simulink model "unfinished_total"  (Simulink 7.9)
settings: Solver=ode3  StartTime=0.0  StopTime=100.0  RelTol=1e-3
undefined symbols (not defined in the file or in its folder): DiscIntNeverNeededParam
libraries: dspsrcs4 x1, simulink x1
settings Model: Creator=dAN  LastModifiedBy=dAN

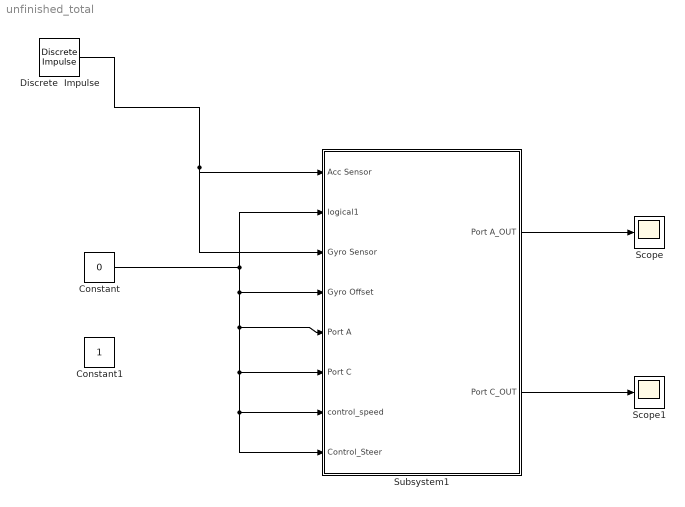
== system unfinished_total ==
  Constant : Constant  Value=0
  Constant1 : Constant
  Discrete  Impulse : dspsrcs4/Discrete  Impulse  Delay=5  SampleTime=1  FrameSample=1  dataType=double  isSigned=on  wordLen=16  udDataType=sfix(16)  fracBitsMode=Best precision  numFracBits=15  OutDataTypeStr=double  LastOutDataTypeStr=double
  Scope : Scope
  Scope1 : Scope
      settings: TimeRange=10
  Subsystem1 : Subsystem
  wires:
  Subsystem1/2(Port C_OUT) -> Scope1/1
  Subsystem1/1(Port A_OUT) -> Scope/1
  Constant/1 -> Subsystem1/4(Gyro Offset), Subsystem1/5(Port A), Subsystem1/7(control_speed), Subsystem1/8(Control_Steer), Subsystem1/6(Port C), Subsystem1/2(logical1)
  Discrete  Impulse/1 -> Subsystem1/1(Acc Sensor), Subsystem1/3(Gyro Sensor)

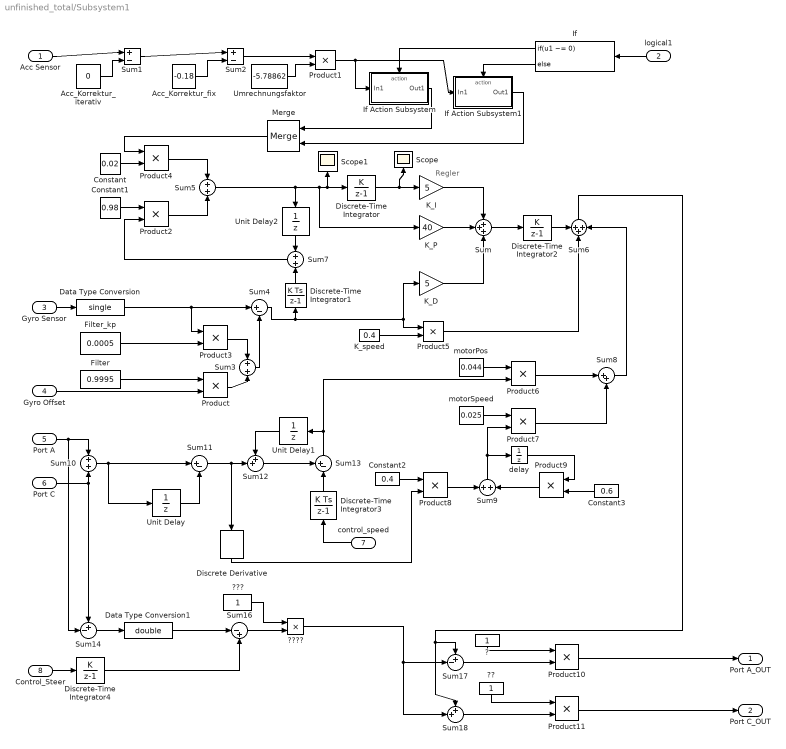
== system unfinished_total/Subsystem1 ==
  note: Regler
  Acc Sensor : Inport
  logical1 : Inport  Port=2
  Gyro Sensor : Inport  Port=3
  Gyro Offset : Inport  Port=4
  Port A : Inport  Port=5
  Port C : Inport  Port=6
  control_speed : Inport  Port=7
  Control_Steer : Inport  Port=8
  "?" : Constant
  "??" : Constant
  "???" : Constant
  "????" : Product  RndMeth=Zero
  Acc_Korrektur_fix : Constant  Value=-0.18
  Acc_Korrektur_iterativ : Constant  Value=0
  Constant : Constant  Value=0.02
  Constant1 : Constant  Value=0.98
  Constant2 : Constant  Value=0.4
  Constant3 : Constant  Value=0.6
  Data Type Conversion : DataTypeConversion  OutDataTypeStr=single  ConvertRealWorld=Stored Integer (SI)
  Data Type Conversion1 : DataTypeConversion  OutDataTypeStr=double  ConvertRealWorld=Stored Integer (SI)
  Discrete Derivative : simulink/Discrete/Discrete Derivative  gainval=1.0  ICPrevScaledInput=0.0  InputProcessing=Inherited  OutMin=[]  OutMax=[]  OutDataType=fixdt(1, 16)  OutScaling=2^-10  DoSatur=off
  Discrete-Time Integrator : DiscreteIntegrator  IntegratorMethod=Accumulation: Forward Euler  ICPrevOutput=DiscIntNeverNeededParam  ICPrevScaledInput=DiscIntNeverNeededParam
  Discrete-Time Integrator1 : DiscreteIntegrator  ICPrevOutput=DiscIntNeverNeededParam  ICPrevScaledInput=DiscIntNeverNeededParam
  Discrete-Time Integrator2 : DiscreteIntegrator  IntegratorMethod=Accumulation: Forward Euler  ICPrevOutput=DiscIntNeverNeededParam  ICPrevScaledInput=DiscIntNeverNeededParam
  Discrete-Time Integrator3 : DiscreteIntegrator  ICPrevOutput=DiscIntNeverNeededParam  ICPrevScaledInput=DiscIntNeverNeededParam
  Discrete-Time Integrator4 : DiscreteIntegrator  IntegratorMethod=Accumulation: Forward Euler  ICPrevOutput=DiscIntNeverNeededParam  ICPrevScaledInput=DiscIntNeverNeededParam
  Filter : Constant  Value=0.9995
  Filter_kp : Constant  Value=0.0005
  If : If  IfExpression=u1 ~= 0
  If Action Subsystem : Subsystem  TreatAsAtomicUnit=on
  If Action Subsystem1 : Subsystem  TreatAsAtomicUnit=on
  K_D : Gain  Gain=5
  K_I : Gain  Gain=5
  K_P : Gain  Gain=40
  K_speed : Constant  Value=0.4
  Merge : Merge
  Product{,1..11} (12 alike) : Product  RndMeth=Zero
  Scope : Scope
      settings: SaveName=ScopeData2
  Scope1 : Scope
      settings: SaveName=ScopeData3
  Sum : Sum  Inputs=+++
  Sum{1..2,4,11} (4 alike) : Sum  Inputs=|+-
  Sum{3,5,7,9..10} (5 alike) : Sum  Inputs=+|+
  Sum12 : Sum  Inputs=++|
  Sum13 : Sum  Inputs=+-|
  Sum14 : Sum  Inputs=+-|
  Sum16 : Sum  Inputs=|-+
  Sum17 : Sum  Inputs=+-|
  Sum18 : Sum  Inputs=++|
  Sum6 : Sum  Inputs=+++
  Sum8 : Sum  Inputs=|++
  Umrechnungsfaktor : Constant  Value=-5.78862
  Unit Delay : UnitDelay  SampleTime=-1
  Unit Delay1 : UnitDelay  SampleTime=-1
  Unit Delay2 : UnitDelay  SampleTime=-1
  delay : UnitDelay  SampleTime=-1
  motorPos : Constant  Value=0.044
  motorSpeed : Constant  Value=0.025
  Port A_OUT : Outport
  Port C_OUT : Outport  Port=2
  wires:
  K_I/1 -> Sum/1
  K_P/1 -> Sum/2
  K_D/1 -> Sum/3
  Discrete-Time Integrator/1 -> K_I/1, Scope/1
  Gyro Offset/1 -> Product/2
  Filter/1 -> Product/1
  Acc Sensor/1 -> Sum1/1
  Acc_Korrektur_iterativ/1 -> Sum1/2
  Acc_Korrektur_fix/1 -> Sum2/2
  Sum1/1 -> Sum2/1
  Umrechnungsfaktor/1 -> Product1/2
  Sum2/1 -> Product1/1
  Gyro Sensor/1 -> Data Type Conversion/1
  Data Type Conversion/1 -> Product3/1, Sum4/1
  Filter_kp/1 -> Product3/2
  Product3/1 -> Sum3/1
  Product/1 -> Sum3/2
  Sum3/1 -> Sum4/2
  Constant/1 -> Product4/2
  Constant1/1 -> Product2/1
  Product4/1 -> Sum5/1
  Product2/1 -> Sum5/2
  Sum7/1 -> Product2/2
  Sum5/1 -> K_P/1, Discrete-Time Integrator/1, Scope1/1, Unit Delay2/1
  Sum/1 -> Discrete-Time Integrator2/1
  K_speed/1 -> Product5/2
  Discrete-Time Integrator2/1 -> Sum6/1
  Product5/1 -> Sum6/2
  Sum8/1 -> Sum6/3
  motorPos/1 -> Product6/1
  Product6/1 -> Sum8/1
  Product7/1 -> Sum8/2
  motorSpeed/1 -> Product7/1
  Product8/1 -> Sum9/1
  Sum9/1 -> Product7/2, delay/1
  Port A/1 -> Sum10/1, Sum14/2
  Port C/1 -> Sum10/2, Sum14/1
  Sum10/1 -> Sum11/1, Unit Delay/1
  Unit Delay/1 -> Sum11/2
  Sum13/1 -> Product6/2, Unit Delay1/1
  Sum12/1 -> Sum13/1
  Sum11/1 -> Sum12/2, Discrete Derivative/1
  Discrete-Time Integrator3/1 -> Sum13/2
  control_speed/1 -> Discrete-Time Integrator3/1
  Product9/1 -> Sum9/2
  Constant3/1 -> Product9/2
  Constant2/1 -> Product8/1
  Discrete Derivative/1 -> Product8/2
  Sum14/1 -> Data Type Conversion1/1
  Control_Steer/1 -> Discrete-Time Integrator4/1
  Data Type Conversion1/1 -> Sum16/1
  Sum16/1 -> "????"/2
  "???"/1 -> "????"/1
  Sum17/1 -> Product10/2
  "?"/1 -> Product10/1
  Product10/1 -> Port A_OUT/1
  "??"/1 -> Product11/1
  Product11/1 -> Port C_OUT/1
  Sum18/1 -> Product11/2
  "????"/1 -> Sum17/2, Sum18/2
  Discrete-Time Integrator4/1 -> Sum16/2
  Sum6/1 -> Sum17/1, Sum18/1
  Unit Delay1/1 -> Sum12/1
  delay/1 -> Product9/1
  Product1/1 -> If Action Subsystem/1(In1), If Action Subsystem1/1(In1)
  If/1 -> If Action Subsystem/Action
  logical1/1 -> If/1
  If/2 -> If Action Subsystem1/Action
  If Action Subsystem/1(Out1) -> Merge/1
  If Action Subsystem1/1(Out1) -> Merge/2
  Merge/1 -> Product4/1
  Sum4/1 -> Discrete-Time Integrator1/1, K_D/1, Product5/1
  Discrete-Time Integrator1/1 -> Sum7/2
  Unit Delay2/1 -> Sum7/1

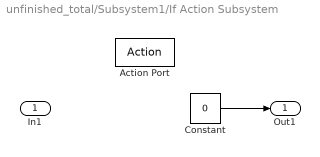
== system unfinished_total/Subsystem1/If Action Subsystem ==
  In1 : Inport
  Action Port : ActionPort  ActionType=then
  Constant : Constant  Value=0
  Out1 : Outport
  wires:
  Constant/1 -> Out1/1

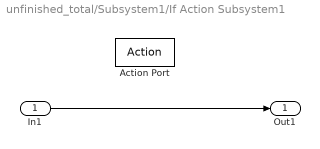
== system unfinished_total/Subsystem1/If Action Subsystem1 ==
  In1 : Inport
  Action Port : ActionPort  ActionType=else
  Out1 : Outport
  wires:
  In1/1 -> Out1/1
